simulink model "ODE1"  (R2018a)
settings: Solver=VariableStepAuto  StartTime=0.0  StopTime=1  RelTol=1e-3
settings Model: Creator=Abhishek Srivastava  LastModifiedBy=Abhishek Srivastava

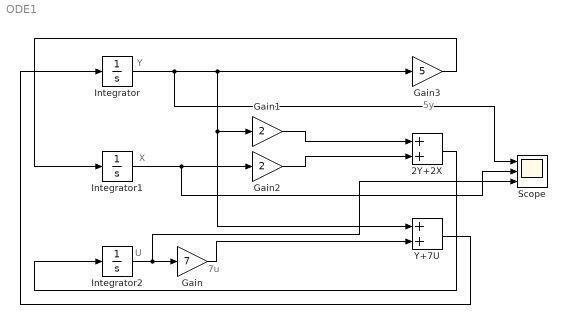
== system ODE1 ==
  note: 5y
  note: 7u
  note: Y
  note: X
  note: U
  2Y+2X : Sum
  Gain : Gain  Gain=7
  Gain1 : Gain  Gain=2
  Gain2 : Gain  Gain=2
  Gain3 : Gain  Gain=5
  Integrator : Integrator  InitialCondition=1
  Integrator1 : Integrator  InitialCondition=2
  Integrator2 : Integrator
  Scope : Scope  NumInputPorts=3
  Y+7U : Sum
  wires:
  Gain/1 -> Y+7U/2
  Integrator/1 -> Scope/1, Gain3/1, Gain1/1, Y+7U/1
  Gain1/1 -> 2Y+2X/1
  Integrator1/1 -> Scope/2, Gain2/1
  Gain2/1 -> 2Y+2X/2
  Gain3/1 -> Integrator1/1
  2Y+2X/1 -> Integrator2/1
  Y+7U/1 -> Integrator/1
  Integrator2/1 -> Scope/3, Gain/1
